simulink model "SP_nonlinear_LQR"  (R2016b)
settings: Solver=ode4  StartTime=0.0  StopTime=100  FixedStep=0.001  RelTol=1e-3
values from neighbouring files (symbols this model uses):
  K = lqr(P_sp,Q,R)    [SP_LQG_controller_design.m]
  Ke_sp = K_bar(:,1)    [SP_LQG_controller_design.m]    (also in controller_parameter.mat = -14.1421356237)
  Kx_sp = K_bar(:,2:end)    [SP_LQG_controller_design.m]    (also in controller_parameter.mat = [-9.4028503548 -29.2130812278])
undefined symbols (not defined in the file or in its folder): An, Aqw, Asp1, Bn, Bqw, Bsp1, Cn, Cqw, Csp1, Kn, lin_sys, Nu, Nu_inv, Nx, Ny, op
libraries: aerolibatmos2 x10, aerolib3dof2 x1, aerolib6dof2 x1, aerolibasang x1
(part 1 of 7)
settings Model: Creator=whn  LastModifiedBy=whn

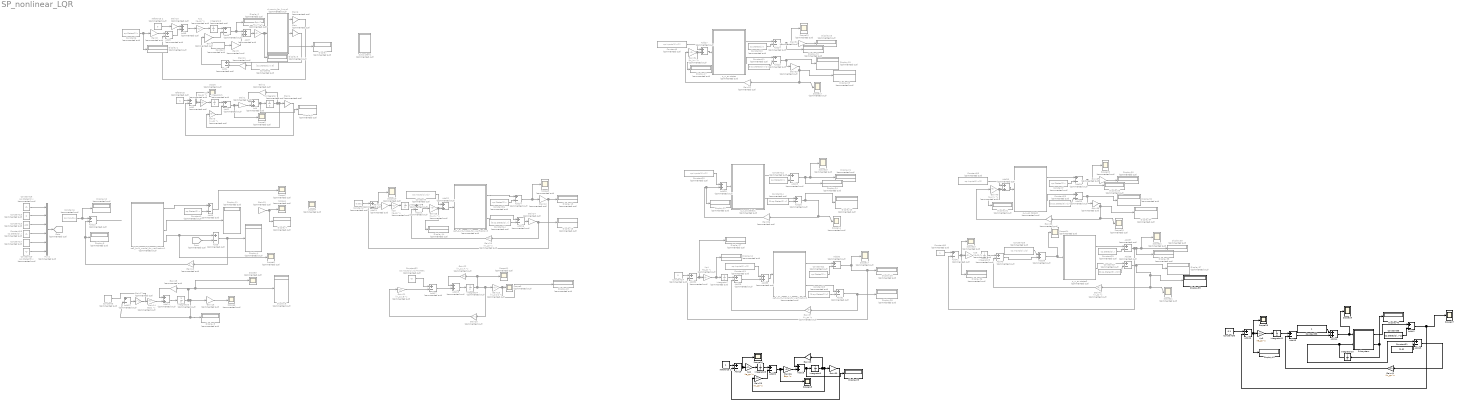
== system SP_nonlinear_LQR ==
  Add{,5,7,11,15,22,27..28,33,36,39} (11 alike) : Sum  Commented=on
  Add{1..4,6,8..10,12..14,16..17,21,23..26,29..32,34..35,37..38,40..41} (28 alike) : Sum  Commented=on  Inputs=+-
  Add18 : Sum
  Add{19..20,42..43,45..46} (6 alike) : Sum  Inputs=+-
  Add44 : Sum
  Constant : Constant  Commented=on  Value=op.Inputs.u(2)
  Constant{1,6..7,10,12,16,18,22,29,34} (10 alike) : Constant  Commented=on  Value=op.States(2).x
  Constant11 : Constant  Commented=on  Value=[0;op.States(3).x(2)]
  Constant13 : Constant  Commented=on  Value=400
  Constant14 : Constant  Commented=on  Value=[0;op.States(2).x]
  Constant15 : Constant  Commented=on  Value=0
  Constant17 : Constant  Commented=on  Value=10000
  Constant19 : Constant  Commented=on  Value=op.States(5).x
  Constant2 : Constant  Commented=on  Value=[op.States(2).x;0]
  Constant{3,9,20..21,26,28} (6 alike) : Constant  Commented=on  Value=op.Inputs(1).u(2)
  Constant23 : Constant  Commented=on  Value=[0;op.States(2).x]
  Constant24 : Constant  Commented=on  Value=0
  Constant25 : Constant  Commented=on  Value=[0;op.States(3).x(2)]
  Constant27 : Constant  Commented=on  Value=[0;op.States(3).x(2)]
  Constant30 : Constant  Commented=on
  Constant31 : Constant  Value=[1;0]  VectorParams1D=off
  Constant32 : Constant  Commented=on  Value=op.Inputs(1).u(2)*0.0001
  Constant33 : Constant
  Constant35 : Constant  Value=op.States(2).x*10
  Constant36 : Constant  Value=0.1
  Constant4 : Constant  Commented=on  Value=op.Inputs.u
  Constant44 : Constant  Commented=on  Value=[0;op.States(2).x]
  Constant5 : Constant  Commented=on  Value=[0 0.001]
  Constant8 : Constant  Commented=on  Value=0.001
  Display{,1..28,30..38} (38 alike) : Display  Commented=on
  Display{29,39..41} (4 alike) : Display
  From : From  Commented=on  GotoTag=states0
  Gain{,11,13,24,33,39} (6 alike) : Gain  Commented=on  Gain=Nx  Multiplication=Matrix(K*u)
  Gain1 : Gain  Commented=on  Gain=Bn  Multiplication=Matrix(K*u)
  Gain{6,8,10,12,27,31,35} (7 alike) : Gain  Commented=on  Gain=Ny  Multiplication=Matrix(K*u)
  Gain14 : Gain  Commented=on  Gain=Bsp1  Multiplication=Matrix(K*u)
  Gain15 : Gain  Commented=on  Gain=Asp1  Multiplication=Matrix(K*u)
  Gain16 : Gain  Commented=on  Gain=Csp1  Multiplication=Matrix(K*u)
  Gain17 : Gain  Commented=on  Gain=K  Multiplication=Matrix(K*u)
  Gain18 : Gain  Commented=on  Gain=K  Multiplication=Matrix(K*u)
  Gain{3,5,19,37,42} (5 alike) : Gain  Commented=on  Gain=Kx_sp  Multiplication=Matrix(K*u)
  Gain2 : Gain  Commented=on  Gain=An  Multiplication=Matrix(K*u)
  Gain20 : Gain  Commented=on  Gain=K  Multiplication=Matrix(K*u)
  Gain21 : Gain  Commented=on  Gain=lin_sys.B  Multiplication=Matrix(K*u)
  Gain22 : Gain  Commented=on  Gain=lin_sys.A  Multiplication=Matrix(K*u)
  Gain23 : Gain  Commented=on  Gain=lin_sys.C  Multiplication=Matrix(K*u)
  Gain{7,25,34,40} (4 alike) : Gain  Commented=on  Gain=Nu_inv  Multiplication=Matrix(K*u)
  Gain26 : Gain  Gain=Bqw  Multiplication=Matrix(K*u)
  Gain28 : Gain  Gain=Aqw  Multiplication=Matrix(K*u)
  Gain29 : Gain  Gain=Kx_sp  Multiplication=Matrix(K*u)
  Gain30 : Gain  Gain=Cqw  Multiplication=Matrix(K*u)
  Gain32 : Gain  Commented=on  Gain=-Kn  Multiplication=Matrix(K*u)
  Gain36 : Gain  Commented=on  Gain=-K  Multiplication=Matrix(K*u)
  Gain38 : Gain  Commented=on  Gain=-Kn  Multiplication=Matrix(K*u)
  Gain4 : Gain  Commented=on  Gain=Cn  Multiplication=Matrix(K*u)
  Gain41 : Gain  Gain=Kx_sp  Multiplication=Matrix(K*u)
  Gain9 : Gain  Commented=on  Gain=Nu  Multiplication=Matrix(K*u)
  Goto : Goto  Commented=on  GotoTag=states0
  Integrator{,1..4,6..7,9} (8 alike) : Integrator  Commented=on
  Integrator10 : Integrator  InitialCondition=[1;0]
  Integrator11 : Integrator
  Integrator5 : Integrator
  Integrator8 : Integrator
  Kp{,1,3..4,6} (5 alike) : Gain  Commented=on  Gain=Ke_sp  Multiplication=Matrix(K*u)
  Kp2 : Gain  Gain=Ke_sp  Multiplication=Matrix(K*u)
  Kp5 : Gain  Gain=Ke_sp  Multiplication=Matrix(K*u)
  Mux2 : Mux  Commented=on  Inputs=6
  Scope{,1..15,17,19..24} (23 alike) : Scope  Commented=on
  Scope{16,18,27..29} (5 alike) : Scope
  Subsystem : Subsystem
  Subsystem1 : Subsystem  Commented=on
  dynamic_for_linsys1 : Subsystem  Commented=on
  q_w_as states : Subsystem  Commented=on
  q_w_as states1 : Subsystem  Commented=on
  q_w_as states2 : Subsystem  Commented=on
  q_w_as states3 : Subsystem  Commented=on
  "reference " : Constant  Commented=on
  reference 1 : Constant
  reference 2 : Constant  Commented=on  Value=0
  sefl_built_model_for_verification1 : Subsystem  Commented=on
  sefl_built_model_for_verification2 : Subsystem  Commented=on
  sefl_built_model_for_verification3 : Subsystem  Commented=on
  wires:
  Gain1/1 -> Add/2
  Add/1 -> Display5/1, Integrator/1
  Gain2/1 -> Add/1
  Gain3/1 -> Add2/2
  Integrator/1 -> Gain3/1, Gain4/1, Gain2/1
  Constant/1 -> Gain9/1
  Gain5/1 -> Add6/2
  Add7/1 -> Gain7/1
  Constant2/1 -> Gain11/1
  Add4/1 -> Gain5/1
  Gain4/1 -> Add1/2
  Add1/1 -> Scope/1, Kp/1
  Kp/1 -> Integrator1/1
  "reference "/1 -> Add1/1
  Integrator1/1 -> Add2/1
  Add2/1 -> Scope2/1, Gain1/1
  Kp1/1 -> Integrator2/1
  Integrator2/1 -> Add6/1
  Add6/1 -> Display2/1, Add7/1
  Constant6/1 -> Display1/1, Gain8/1
  Gain6/1 -> Add3/2
  reference 2/1 -> Gain10/1
  Add3/1 -> Add5/2
  Add5/1 -> Kp1/1
  dynamic_for_linsys1/3(states_dot) -> Display/1
  dynamic_for_linsys1/2("states ") -> Gain/1
  Gain/1 -> Add4/1
  dynamic_for_linsys1/1(output_alpha) -> Gain6/1
  Gain7/1 -> Display3/1, dynamic_for_linsys1/1(In1)
  Gain8/1 -> Add3/1
  Gain9/1 -> Add7/2
  Gain10/1 -> Add5/1
  Gain11/1 -> Add4/2
  sefl_built_model_for_verification1/1(Out5) -> Add8/1
  Constant4/1 -> Display10/1, Add13/1
  Constant1/1 -> Add8/2
  Add8/1 -> Scope7/1
  Add9/1 -> Gain18/1, Display4/1
  sefl_built_model_for_verification1/4(states) -> Add9/1, Scope8/1
  Gain13/1 -> Scope1/1, Display7/1
  Gain14/1 -> Add11/2
  Add11/1 -> Integrator3/1
  Gain15/1 -> Add11/1
  Integrator3/1 -> Display8/1, Add12/2, Gain16/1, Scope3/1, Display6/1, Gain15/1
  Gain18/1 -> Add13/2, Display9/1
  Add12/1 -> Gain17/1
  Constant5/1 -> Gain14/1
  Gain17/1 -> ?
  Gain16/1 -> Scope6/1
  Constant13/1 -> Mux2/3
  Constant16/1 -> Mux2/1
  Constant15/1 -> Mux2/2
  Constant18/1 -> Mux2/4
  Constant17/1 -> Mux2/5
  Constant19/1 -> Mux2/6
  Mux2/1 -> Goto/1
  From/1 -> Add9/2
  Add13/1 -> ?
  sefl_built_model_for_verification1/3(states_dot) -> Display11/1
  Add15/1 -> Integrator4/1
  Gain22/1 -> Add15/1
  Integrator4/1 -> Gain20/1, Gain23/1, Scope11/1, Gain22/1
  Constant32/1 -> Add17/1
  Constant3/1 -> Add22/1
  sefl_built_model_for_verification3/1(alpha_for_tracking) -> Add14/1
  Constant34/1 -> Add14/2
  Add14/1 -> Scope5/1, Gain12/1
  Gain23/1 -> Display18/1, Scope9/1
  sefl_built_model_for_verification3/2(states_q_w) -> Add16/1
  Constant44/1 -> Add16/2
  Gain24/1 -> Gain19/1, Display15/1
  Gain19/1 -> Add10/2
  Gain20/1 -> Gain21/1
  Gain21/1 -> Add17/2
  Add17/1 -> Add15/2
  Add16/1 -> Gain24/1
  Gain25/1 -> Display14/1, Add22/2
  Integrator6/1 -> Add10/1
  Kp3/1 -> Integrator6/1
  Add21/1 -> Scope10/1, Gain27/1
  Gain27/1 -> Kp3/1
  Gain12/1 -> Display13/1, Add21/2  "tracking design for normalized system"
  Constant8/1 -> Add21/1
  Add10/1 -> Gain25/1
  Add22/1 -> sefl_built_model_for_verification3/1(In1)
  Constant9/1 -> Add27/1
  q_w_as states/1(alpha_for_tracking) -> Add24/1
  Constant10/1 -> Add24/2
  Add24/1 -> Display20/1, Scope13/1, Gain31/1
  q_w_as states/2(states_q_w) -> Add25/1
  Constant11/1 -> Add25/2
  Gain33/1 -> Display25/1, Scope12/1, Gain32/1  "normalized system for lqr verification"
  Gain32/1 -> Gain34/1
  Add25/1 -> Gain33/1, Display19/1
  Gain34/1 -> Display17/1, Add27/2
  Gain31/1 -> Display16/1
  Add27/1 -> q_w_as states/1(In1)
  Constant20/1 -> Add28/1
  q_w_as states1/1(alpha_for_tracking) -> Add23/1
  Constant12/1 -> Add23/2
  q_w_as states1/2(states_q_alpha) -> Add26/1
  Constant14/1 -> Add26/2
  Add26/1 -> Scope14/1, Gain36/1, Display23/1  "non_normalized system for lqr verification"
  Gain36/1 -> Add28/2, Display22/1
  Add23/1 -> Display24/1, Display21/1, Scope15/1
  Add28/1 -> q_w_as states1/1(In1)
  Constant21/1 -> Add33/1
  sefl_built_model_for_verification2/1(alpha_for_tracking) -> Add30/1
  Constant22/1 -> Add30/2
  sefl_built_model_for_verification2/2(states_q_alpha) -> Add31/1
  Constant23/1 -> Add31/2
  Add31/1 -> Gain37/1, Display28/1
  Gain37/1 -> Add29/2
  Add29/1 -> Add33/2
  Integrator7/1 -> Add29/1
  Kp4/1 -> Display12/1, Integrator7/1
  Add32/1 -> Display27/1, Kp4/1
  Add30/1 -> Display26/1, Add32/2, Scope17/1  "non-normalized system for tracking"
  Constant24/1 -> Add32/1
  Add33/1 -> sefl_built_model_for_verification2/1(In1)
  Gain26/1 -> Add18/2
  Add18/1 -> Integrator5/1, Display29/1
  Gain28/1 -> Add18/1
  Gain29/1 -> Add20/2
  Integrator5/1 -> Gain28/1, Gain30/1, Gain29/1
  Gain30/1 -> Add19/2
  Add19/1 -> Kp2/1, Scope16/1
  Kp2/1 -> Integrator8/1
  reference 1/1 -> Add19/1
  Integrator8/1 -> Add20/1
  Add20/1 -> Gain26/1, Scope18/1
  Constant26/1 -> Add36/1
  q_w_as states2/1(alpha_for_tracking) -> Add34/1
  Constant7/1 -> Add34/2
  Add34/1 -> Display33/1, Scope20/1, Gain35/1
  q_w_as states2/2(states_q_w) -> Add35/1
  Constant25/1 -> Add35/2
  Gain39/1 -> Display34/1, Scope19/1, Gain38/1  "normalized system for lqr verification_q_w"
  Gain38/1 -> Gain40/1
  Add35/1 -> Gain39/1, Display32/1
  Gain40/1 -> Display31/1, Add36/2
  Gain35/1 -> Display30/1
  Add36/1 -> q_w_as states2/1(In1)
  Constant28/1 -> Add39/1
  q_w_as states3/1(alpha_for_tracking) -> Add37/1
  Constant29/1 -> Add37/2
  q_w_as states3/2(states_q_w) -> Add38/1
  Constant27/1 -> Add38/2
  Add38/1 -> Display39/1, Scope21/1, Gain42/1, Display37/1  "non_normalized system for lqr verification_q_W"
  Add39/1 -> q_w_as states3/1(In1), Scope24/1
  Gain42/1 -> Add40/2
  Add40/1 -> Add39/2
  Integrator9/1 -> Add40/1
  Kp6/1 -> Integrator9/1
  Add41/1 -> Display36/1, Scope23/1, Kp6/1
  Add37/1 -> Display38/1, Display35/1, Scope22/1, Add41/2  "non-normalized system for tracking"
  Constant30/1 -> Add41/1
  Subsystem/2(Xdotbar) -> Integrator10/1, Display40/1
  Integrator10/1 -> Subsystem/2(Xbar), Add43/1
  Constant33/1 -> Add44/1
  Subsystem/1(Ybar) -> Add42/1
  Constant35/1 -> Add42/2
  Constant31/1 -> Add43/2
  Add43/1 -> Gain41/1
  Add44/1 -> Scope29/1, Subsystem/1(Ubar)
  Gain41/1 -> Add45/2
  Add45/1 -> Add44/2
  Integrator11/1 -> Add45/1
  Kp5/1 -> Integrator11/1
  Add46/1 -> Display41/1, Scope28/1, Kp5/1
  Add42/1 -> Scope27/1, Add46/2  "non-normalized system for tracking"
  Constant36/1 -> Add46/1

== system SP_nonlinear_LQR/Subsystem ==
  Ubar : Inport
  Xbar : Inport  Port=2
  Constant2 : Constant  Value=10
  Constant24 : Constant
  Constant25 : Constant  Value=op.States(3).x(2)
  Constant29 : Constant  Value=op.Inputs(1).u(2)
  Demux3 : Demux  Outputs=2
  Mux3 : Mux  Inputs=2
  Product : Product  Inputs=*/
  Product1 : Product
  Product2 : Product
  Product3 : Product
  sefl_built_model : Subsystem
  Ybar : Outport
  Xdotbar : Outport  Port=2
  wires:
  Mux3/1 -> Product/2, Product3/1
  Xbar/1 -> Product3/2
  sefl_built_model/1(alpha_for_tracking) -> Product1/1
  Product1/1 -> Ybar/1
  Product3/1 -> Demux3/1
  sefl_built_model/2(states_dot) -> Product/1
  Constant29/1 -> Product2/1
  Constant2/1 -> Product1/2
  Product2/1 -> sefl_built_model/1(In1)
  Product/1 -> Xdotbar/1
  Demux3/1 -> sefl_built_model/2(w)
  Constant25/1 -> Mux3/1
  Constant24/1 -> Mux3/2
  Demux3/2 -> sefl_built_model/3(q)
  Ubar/1 -> Product2/2

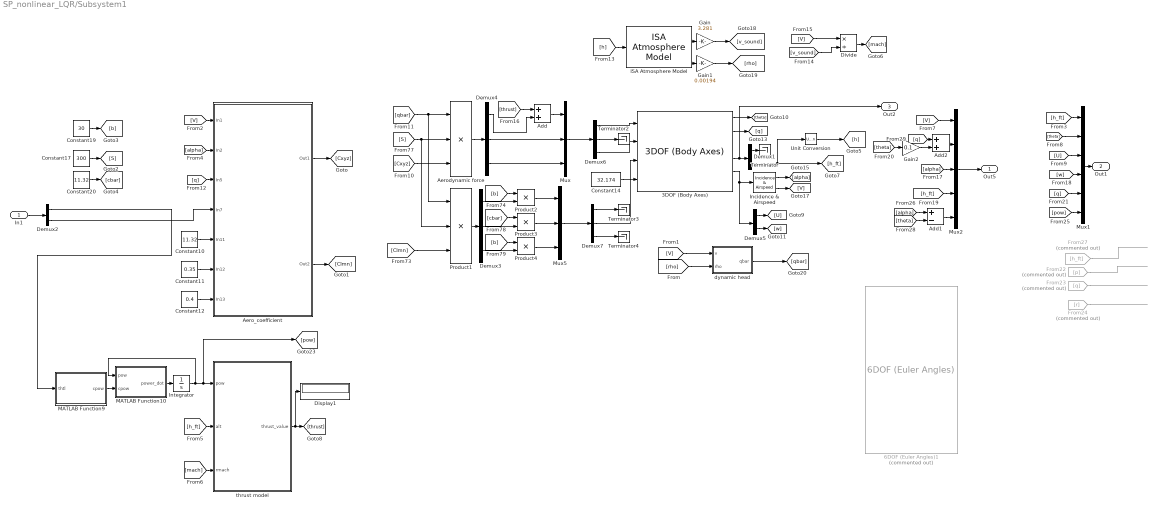
== system SP_nonlinear_LQR/Subsystem1 ==
  In1 : Inport
  3DOF (Body Axes) : aerolib3dof2/3DOF (Body Axes)  units=English (Velocity in ft/s)  mtype=Fixed  v_ini=400  theta_ini=op.States(2).x  alpha_ini=op.States(2).x  q_ini=0  pos_ini=[0 10000]  mass=1/1.57e-3  mass_e=0.5  mass_f=3.0  Iyy=55814  Iyy_e=0.5  Iyy_f=3.0  g_in=External  g=9.81  vre_flag=on
  6DOF (Euler Angles)1 : aerolib6dof2/6DOF (Euler Angles)  Commented=on  units=English (Velocity in ft/s)  mtype=Fixed  rep=Euler Angles  xme_0=[0 0 10000]  Vm_0=[294.1676 0.0066 58.8681]  eul_0=[0 0.1975 0]  pm_0=[0 0 0]  mass_0=1/1.57e-3  mass_e=0.5  mass_f=2.0  inertia=[9496 0 -982;0 55814 0;0 0 63100]  inertia_e=eye(3)  inertia_f=2*eye(3)  k_quat=1.0  vre_flag=on
  Add : Sum
  Add1 : Sum  Inputs=+-
  Add2 : Sum
  Aero_coefficient : Subsystem
      mask Display:
      | port_label('input', 1, 'vt')
      | port_label('input', 2, 'alpha')
      | 
      | port_label('input', 3, 'q')
      | 
      | port_label('input', 4, 'el')
      | 
      | 
      | 
      | port_label('input', 5, 'cbar')
      | port_label('input', 6, 'xcgr')
      | port_label('input', 7, 'xcg')
      | port_label('output', 1, 'Cxz')
      | port_label('output', 2, 'Cm')
  "Aerodynamic force " : Product  Inputs=3
  Constant10 : Constant  Value=11.32
  Constant11 : Constant  Value=0.35
  Constant12 : Constant  Value=0.4
  Constant14 : Constant  Value=32.174
  Constant17 : Constant  Value=300
  Constant19 : Constant  Value=30
  Constant20 : Constant  Value=11.32
  Demux1 : Demux  Outputs=2
  Demux2 : Demux  Outputs=2
  Demux{3..4,6..7} (4 alike) : Demux  Outputs=3
  Demux5 : Demux  Outputs=2
  Display1 : Display
  Divide : Product  Inputs=*/
  From22 : From  Commented=on  GotoTag=p
  From23 : From  Commented=on  GotoTag=q
  From24 : From  Commented=on  GotoTag=r
  From27 : From  Commented=on  GotoTag=h_ft
  Gain : Gain  Gain=3.281
  Gain1 : Gain  Gain=0.00194
  Gain2 : Gain  Gain=0.1
  ISA Atmosphere Model : aerolibatmos2/ISA Atmosphere Model  custom=off  g=9.80665  gamma=1.4  R=287.0531  L=0.0065  h_trop=11000  h_strat=20000  rho0=1.225  P0=101325  T0=288.15  h0=0
  Incidence & Airspeed : aerolibasang/Incidence  & Airspeed
  Integrator : Integrator  InitialCondition=op.states(5).x
  MATLAB Function10 : MATLAB Function  TreatAsAtomicUnit=on
  MATLAB Function9 : MATLAB Function  TreatAsAtomicUnit=on
  Mux : Mux  Inputs=3
  Mux1 : Mux  Inputs=6
  Mux2 : Mux  Inputs=5
  Mux5 : Mux  Inputs=3
  Product1 : Product  Inputs=3
  Product2 : Product
  Product3 : Product
  Product4 : Product
  Terminator{,2..4} (4 alike) : Terminator
  Unit Conversion : UnitConversion
  dynamic head : MATLAB Function  TreatAsAtomicUnit=on
  thrust model : MATLAB Function  TreatAsAtomicUnit=on
  Out5 : Outport
  Out1 : Outport  Port=2
  Out2 : Outport  Port=3
  wires:
  Add2/1 -> Mux2/2
  Gain2/1 -> Add2/2
  [q] -> Add2/1
  [theta] -> Add1/2
  [alpha] -> Add1/1
  Add1/1 -> Mux2/5
  3DOF (Body Axes)/5 -> Demux5/1, Incidence & Airspeed/1
  Mux2/1 -> Out5/1
  Incidence & Airspeed/2 -> [V]
  3DOF (Body Axes)/4 -> Demux1/1, Out2/1
  ISA Atmosphere Model/4 -> Gain1/1
  ISA Atmosphere Model/2 -> Gain/1
  [qbar] -> Product1/1, "Aerodynamic force "/1
  In1/1 -> Demux2/1
  Product4/1 -> Mux5/3
  Constant10/1 -> Aero_coefficient/5(In11)
  Constant11/1 -> Aero_coefficient/6(In12)
  Mux5/1 -> Demux7/1
  Constant17/1 -> [S]
  [q] -> Aero_coefficient/3(In5)
  Gain1/1 -> [rho]
  Product3/1 -> Mux5/2
  Product2/1 -> Mux5/1
  [V] -> Divide/1
  [V] -> dynamic head/1(v)
  Aero_coefficient/1(Out1) -> [Cxyz]
  [rho] -> dynamic head/2(rho)
  Aero_coefficient/2(Out2) -> [Clmn]
  Constant20/1 -> [cbar]
  Constant19/1 -> [b]
  Demux1/2 -> [h_ft], Unit Conversion/1
  [h] -> ISA Atmosphere Model/1
  Demux4/3 -> Mux/3
  Gain/1 -> [v_sound]
  Divide/1 -> [mach]
  Add/1 -> Mux/1
  Demux4/2 -> Mux/2
  [v_sound] -> Divide/2
  Demux4/1 -> Add/2
  Mux/1 -> Demux6/1
  Constant12/1 -> Aero_coefficient/7(In13)
  [alpha] -> Aero_coefficient/2(In2)
  Unit Conversion/1 -> [h]
  dynamic head/1(qbar) -> [qbar]
  thrust model/1(thrust_value) -> Display1/1, [thrust]
  Incidence & Airspeed/1 -> [alpha]
  [h_ft] -> thrust model/2(alt)
  Demux2/2 -> Aero_coefficient/4(In7)
  Demux2/1 -> MATLAB Function9/1(thtl)
  Integrator/1 -> MATLAB Function10/1(pow), [pow], thrust model/1(pow)
  [mach] -> thrust model/3(rmach)
  [alpha] -> Mux2/3
  MATLAB Function10/1(power_dot) -> Integrator/1
  [V] -> Aero_coefficient/1(In1)
  MATLAB Function9/1(cpow) -> MATLAB Function10/2(cpow)
  [thrust] -> Add/1
  Demux3/3 -> Product4/2
  [b] -> Product4/1
  "Aerodynamic force "/1 -> Demux4/1
  [Cxyz] -> "Aerodynamic force "/3
  [S] -> "Aerodynamic force "/2, Product1/2
  [Clmn] -> Product1/3
  [b] -> Product2/1
  Product1/1 -> Demux3/1
  Demux3/1 -> Product2/2
  Demux3/2 -> Product3/2
  [cbar] -> Product3/1
  [theta] -> Gain2/1
  [V] -> Mux2/1
  From27/1 -> ?
  From22/1 -> ?
  From23/1 -> ?
  From24/1 -> ?
  [h_ft] -> Mux2/4
  Demux6/1 -> 3DOF (Body Axes)/1
  Demux6/3 -> 3DOF (Body Axes)/2
  Demux6/2 -> Terminator2/1
  Demux7/2 -> 3DOF (Body Axes)/3
  Demux7/1 -> Terminator3/1
  Demux7/3 -> Terminator4/1
  Demux1/1 -> Terminator/1
  3DOF (Body Axes)/1 -> [theta]
  3DOF (Body Axes)/2 -> [q]
  Constant14/1 -> 3DOF (Body Axes)/4
  [h_ft] -> Mux1/1
  [theta] -> Mux1/2
  Demux5/2 -> [w]
  Demux5/1 -> [U]
  [U] -> Mux1/3
  [w] -> Mux1/4
  [q] -> Mux1/5
  [pow] -> Mux1/6
  Mux1/1 -> Out1/1

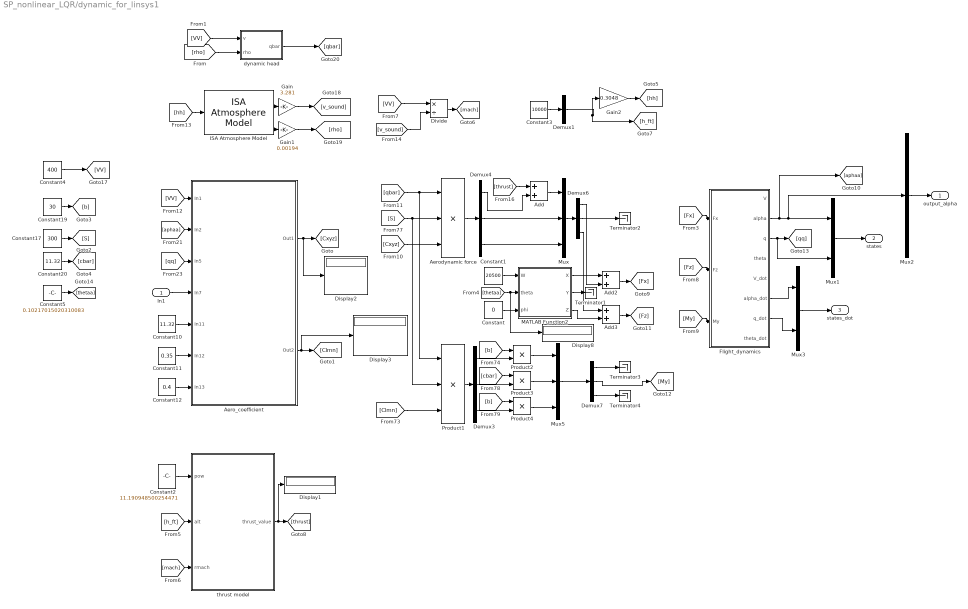
== system SP_nonlinear_LQR/dynamic_for_linsys1 ==
  In1 : Inport
  Add : Sum
  Add2 : Sum
  Add3 : Sum
  Aero_coefficient : Subsystem
      mask Display:
      | port_label('input', 1, 'vt')
      | port_label('input', 2, 'alpha')
      | 
      | port_label('input', 3, 'q')
      | 
      | port_label('input', 4, 'el')
      | 
      | 
      | 
      | port_label('input', 5, 'cbar')
      | port_label('input', 6, 'xcgr')
      | port_label('input', 7, 'xcg')
      | port_label('output', 1, 'Cxz')
      | port_label('output', 2, 'Cm')
  "Aerodynamic force " : Product  Inputs=3
  Constant : Constant  Value=0
  Constant1 : Constant  Value=20500
  Constant10 : Constant  Value=11.32
  Constant11 : Constant  Value=0.35
  Constant12 : Constant  Value=0.4
  Constant17 : Constant  Value=300
  Constant19 : Constant  Value=30
  Constant2 : Constant  Value=11.190948500254471
  Constant20 : Constant  Value=11.32
  Constant3 : Constant  Value=10000
  Constant4 : Constant  Value=400
  Constant5 : Constant  Value=0.10217015020310083
  Demux1 : Demux  Outputs=1
  Demux{3..4,6..7} (4 alike) : Demux  Outputs=3
  Display{1..3,8} (4 alike) : Display
  Divide : Product  Inputs=*/
  Flight_dynamics : Subsystem
  Gain : Gain  Gain=3.281
  Gain1 : Gain  Gain=0.00194
  Gain2 : Gain  Gain=0.3048
  ISA Atmosphere Model : aerolibatmos2/ISA Atmosphere Model  custom=off  g=9.80665  gamma=1.4  R=287.0531  L=0.0065  h_trop=11000  h_strat=20000  rho0=1.225  P0=101325  T0=288.15  h0=0
  MATLAB Function2 : MATLAB Function  TreatAsAtomicUnit=on
  Mux : Mux  Inputs=3
  Mux1 : Mux  Inputs=2
  Mux2 : Mux  Inputs=1
  Mux3 : Mux  Inputs=2
  Mux5 : Mux  Inputs=3
  Product1 : Product  Inputs=3
  Product2 : Product
  Product3 : Product
  Product4 : Product
  Terminator{1..4} (4 alike) : Terminator
  dynamic head : MATLAB Function  TreatAsAtomicUnit=on
  thrust model : MATLAB Function  TreatAsAtomicUnit=on
  output_alpha : Outport
  "states " : Outport  Port=2
  states_dot : Outport  Port=3
  wires:
  [qq] -> Aero_coefficient/3(In5)
  [aphaa] -> Aero_coefficient/2(In2)
  [VV] -> Aero_coefficient/1(In1)
  Constant5/1 -> [thetaa]
  Flight_dynamics/3(q) -> Mux1/2, [qq]
  Flight_dynamics/2(alpha) -> [aphaa], Mux1/1, Mux2/1
  ISA Atmosphere Model/4 -> Gain1/1
  ISA Atmosphere Model/2 -> Gain/1
  [qbar] -> Product1/1, "Aerodynamic force "/1
  In1/1 -> Aero_coefficient/4(In7)
  Product4/1 -> Mux5/3
  Constant10/1 -> Aero_coefficient/5(In11)
  Constant11/1 -> Aero_coefficient/6(In12)
  Mux5/1 -> Demux7/1
  Constant17/1 -> [S]
  Gain1/1 -> [rho]
  Product3/1 -> Mux5/2
  Product2/1 -> Mux5/1
  [VV] -> Divide/1
  [VV] -> dynamic head/1(v)
  Aero_coefficient/1(Out1) -> Display2/1, [Cxyz]
  [rho] -> dynamic head/2(rho)
  Aero_coefficient/2(Out2) -> Display3/1, [Clmn]
  Constant20/1 -> [cbar]
  Constant19/1 -> [b]
  Demux1/1 -> [h_ft], Gain2/1
  [hh] -> ISA Atmosphere Model/1
  Demux4/3 -> Mux/3
  Gain/1 -> [v_sound]
  Divide/1 -> [mach]
  Add/1 -> Mux/1
  Demux4/2 -> Mux/2
  [v_sound] -> Divide/2
  Demux4/1 -> Add/2
  Mux/1 -> Demux6/1
  Constant12/1 -> Aero_coefficient/7(In13)
  Gain2/1 -> [hh]
  dynamic head/1(qbar) -> [qbar]
  thrust model/1(thrust_value) -> Display1/1, [thrust]
  [h_ft] -> thrust model/2(alt)
  [mach] -> thrust model/3(rmach)
  Constant4/1 -> [VV]
  [thrust] -> Add/1
  Demux3/3 -> Product4/2
  [b] -> Product4/1
  "Aerodynamic force "/1 -> Demux4/1
  [Cxyz] -> "Aerodynamic force "/3
  [S] -> "Aerodynamic force "/2, Product1/2
  [Clmn] -> Product1/3
  [b] -> Product2/1
  Product1/1 -> Demux3/1
  Demux3/1 -> Product2/2
  Demux3/2 -> Product3/2
  [cbar] -> Product3/1
  Demux6/3 -> Add3/1
  Demux6/2 -> Terminator2/1
  Demux7/1 -> Terminator3/1
  Demux7/3 -> Terminator4/1
  Mux2/1 -> output_alpha/1
  Constant1/1 -> MATLAB Function2/1(W)
  [thetaa] -> Display8/1, MATLAB Function2/2(theta)
  Constant/1 -> MATLAB Function2/3(phi)
  MATLAB Function2/1(X) -> Add2/1
  Demux6/1 -> Add2/2
  MATLAB Function2/3(Z) -> Add3/2
  MATLAB Function2/2(Y) -> Terminator1/1
  Add2/1 -> [Fx]
  Add3/1 -> [Fz]
  Demux7/2 -> [My]
  [Fx] -> Flight_dynamics/1(Fx)
  [Fz] -> Flight_dynamics/2(Fz)
  [My] -> Flight_dynamics/3(My)
  Mux1/1 -> "states "/1
  Flight_dynamics/6(alpha_dot) -> Mux3/1
  Flight_dynamics/7(q_dot) -> Mux3/2
  Mux3/1 -> states_dot/1
  Constant2/1 -> thrust model/1(pow)
  Constant3/1 -> Demux1/1

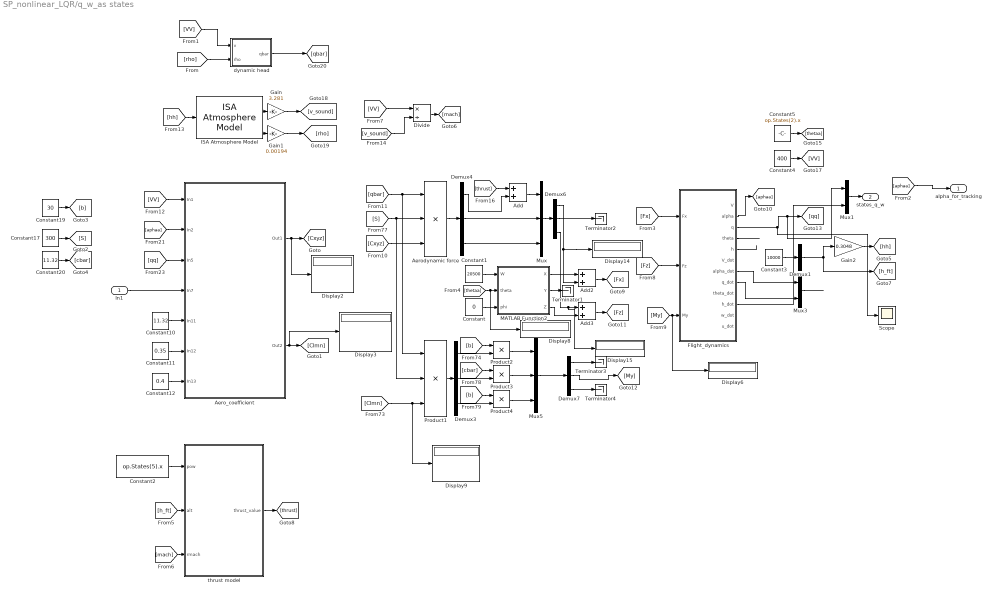
== system SP_nonlinear_LQR/q_w_as states ==
  In1 : Inport
  Add : Sum
  Add2 : Sum
  Add3 : Sum
  Aero_coefficient : Subsystem
      mask Display:
      | port_label('input', 1, 'vt')
      | port_label('input', 2, 'alpha')
      | 
      | port_label('input', 3, 'q')
      | 
      | port_label('input', 4, 'el')
      | 
      | 
      | 
      | port_label('input', 5, 'cbar')
      | port_label('input', 6, 'xcgr')
      | port_label('input', 7, 'xcg')
      | port_label('output', 1, 'Cxz')
      | port_label('output', 2, 'Cm')
  "Aerodynamic force " : Product  Inputs=3
  Constant : Constant  Value=0
  Constant1 : Constant  Value=20500
  Constant10 : Constant  Value=11.32
  Constant11 : Constant  Value=0.35
  Constant12 : Constant  Value=0.4
  Constant17 : Constant  Value=300
  Constant19 : Constant  Value=30
  Constant2 : Constant  Value=op.States(5).x
  Constant20 : Constant  Value=11.32
  Constant3 : Constant  Value=10000
  Constant4 : Constant  Value=400
  Constant5 : Constant  Value=op.States(2).x
  Demux1 : Demux  Outputs=1
  Demux{3..4,6..7} (4 alike) : Demux  Outputs=3
  Display{2..3,6,8..9,14..15} (7 alike) : Display
  Divide : Product  Inputs=*/
  Flight_dynamics : Subsystem
  Gain : Gain  Gain=3.281
  Gain1 : Gain  Gain=0.00194
  Gain2 : Gain  Gain=0.3048
  ISA Atmosphere Model : aerolibatmos2/ISA Atmosphere Model  custom=off  g=9.80665  gamma=1.4  R=287.0531  L=0.0065  h_trop=11000  h_strat=20000  rho0=1.225  P0=101325  T0=288.15  h0=0
  MATLAB Function2 : MATLAB Function  TreatAsAtomicUnit=on
  Mux : Mux  Inputs=3
  Mux1 : Mux  Inputs=2
  Mux3 : Mux  Inputs=2
  Mux5 : Mux  Inputs=3
  Product1 : Product  Inputs=3
  Product2 : Product
  Product3 : Product
  Product4 : Product
  Scope : Scope
  Terminator{1..4} (4 alike) : Terminator
  dynamic head : MATLAB Function  TreatAsAtomicUnit=on
  thrust model : MATLAB Function  TreatAsAtomicUnit=on
  alpha_for_tracking : Outport
  states_q_w : Outport  Port=2
  wires:
  [aphaa] -> alpha_for_tracking/1
  Constant5/1 -> [thetaa]
  Constant4/1 -> [VV]
  Constant3/1 -> Demux1/1
  Constant2/1 -> thrust model/1(pow)
  Flight_dynamics/8(q_dot) -> Mux3/2
  Flight_dynamics/7(alpha_dot) -> Mux3/1
  [qq] -> Aero_coefficient/3(In5)
  [aphaa] -> Aero_coefficient/2(In2)
  [VV] -> Aero_coefficient/1(In1)
  Flight_dynamics/5(h) -> ?
  ISA Atmosphere Model/4 -> Gain1/1
  ISA Atmosphere Model/2 -> Gain/1
  [qbar] -> Product1/1, "Aerodynamic force "/1
  In1/1 -> Aero_coefficient/4(In7)
  Product4/1 -> Mux5/3
  Constant10/1 -> Aero_coefficient/5(In11)
  Constant11/1 -> Aero_coefficient/6(In12)
  Mux5/1 -> Demux7/1
  Constant17/1 -> [S]
  Gain1/1 -> [rho]
  Product3/1 -> Mux5/2
  Product2/1 -> Mux5/1
  [VV] -> Divide/1
  [VV] -> dynamic head/1(v)
  Aero_coefficient/1(Out1) -> Display2/1, [Cxyz]
  [rho] -> dynamic head/2(rho)
  Aero_coefficient/2(Out2) -> [Clmn], Display3/1
  Constant20/1 -> [cbar]
  Constant19/1 -> [b]
  Demux1/1 -> Gain2/1, [h_ft]
  [hh] -> ISA Atmosphere Model/1
  Demux4/3 -> Mux/3
  Gain/1 -> [v_sound]
  Divide/1 -> [mach]
  Add/1 -> Mux/1
  Demux4/2 -> Mux/2
  [v_sound] -> Divide/2
  Demux4/1 -> Add/2
  Mux/1 -> Demux6/1
  Constant12/1 -> Aero_coefficient/7(In13)
  Gain2/1 -> [hh]
  dynamic head/1(qbar) -> [qbar]
  thrust model/1(thrust_value) -> [thrust]
  [h_ft] -> thrust model/2(alt)
  [mach] -> thrust model/3(rmach)
  [thrust] -> Add/1
  Demux3/3 -> Product4/2
  [b] -> Product4/1
  "Aerodynamic force "/1 -> Demux4/1
  [Cxyz] -> "Aerodynamic force "/3
  [S] -> "Aerodynamic force "/2, Product1/2
  [Clmn] -> Display9/1, Product1/3
  [b] -> Product2/1
  Product1/1 -> Demux3/1
  Demux3/1 -> Product2/2
  Demux3/2 -> Product3/2
  [cbar] -> Product3/1
  Demux6/3 -> Display15/1, Add3/1
  Demux6/2 -> Terminator2/1
  Demux7/1 -> Terminator3/1
  Demux7/3 -> Terminator4/1
  Constant1/1 -> MATLAB Function2/1(W)
  [thetaa] -> Display8/1, MATLAB Function2/2(theta)
  Constant/1 -> MATLAB Function2/3(phi)
  MATLAB Function2/1(X) -> Add2/1
  Demux6/1 -> Display14/1, Add2/2
  MATLAB Function2/3(Z) -> Add3/2
  MATLAB Function2/2(Y) -> Terminator1/1
  Add2/1 -> [Fx]
  Add3/1 -> [Fz]
  Demux7/2 -> [My]
  [Fx] -> Flight_dynamics/1(Fx)
  [Fz] -> Flight_dynamics/2(Fz)
  [My] -> Flight_dynamics/3(My), Display6/1
  Mux3/1 -> ?
  Flight_dynamics/2(alpha) -> [aphaa]
  Flight_dynamics/3(q) -> Scope/1, Mux1/1, [qq]
  Flight_dynamics/4(theta) -> ?
  Mux1/1 -> states_q_w/1
  Flight_dynamics/10(h_dot) -> Mux1/2

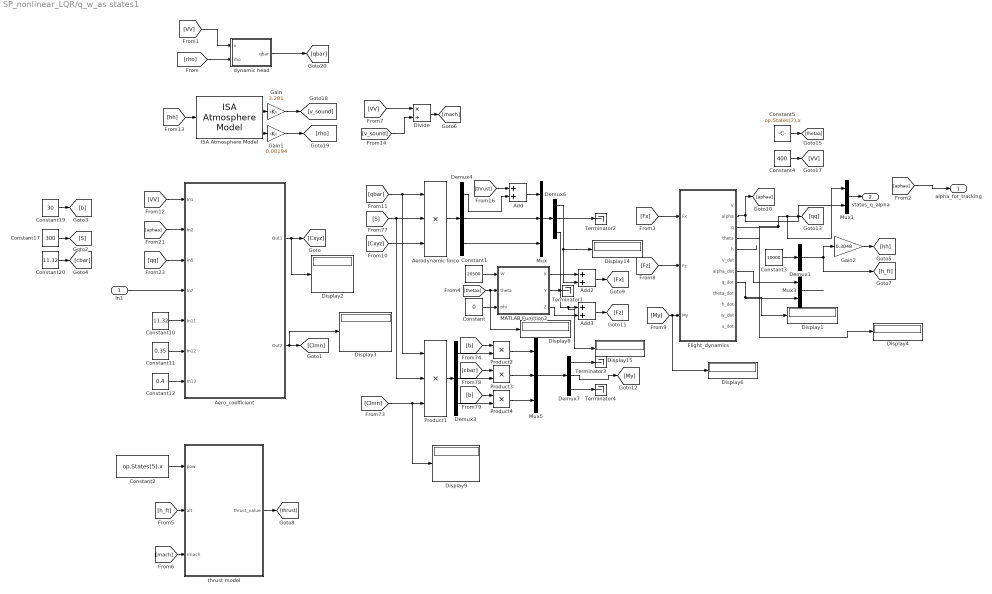
== system SP_nonlinear_LQR/q_w_as states1 ==
  In1 : Inport
  Add : Sum
  Add2 : Sum
  Add3 : Sum
  Aero_coefficient : Subsystem
      mask Display:
      | port_label('input', 1, 'vt')
      | port_label('input', 2, 'alpha')
      | 
      | port_label('input', 3, 'q')
      | 
      | port_label('input', 4, 'el')
      | 
      | 
      | 
      | port_label('input', 5, 'cbar')
      | port_label('input', 6, 'xcgr')
      | port_label('input', 7, 'xcg')
      | port_label('output', 1, 'Cxz')
      | port_label('output', 2, 'Cm')
  "Aerodynamic force " : Product  Inputs=3
  Constant : Constant  Value=0
  Constant1 : Constant  Value=20500
  Constant10 : Constant  Value=11.32
  Constant11 : Constant  Value=0.35
  Constant12 : Constant  Value=0.4
  Constant17 : Constant  Value=300
  Constant19 : Constant  Value=30
  Constant2 : Constant  Value=op.States(5).x
  Constant20 : Constant  Value=11.32
  Constant3 : Constant  Value=10000
  Constant4 : Constant  Value=400
  Constant5 : Constant  Value=op.States(2).x
  Demux1 : Demux  Outputs=1
  Demux{3..4,6..7} (4 alike) : Demux  Outputs=3
  Display{1..4,6,8..9,14..15} (9 alike) : Display
  Divide : Product  Inputs=*/
  Flight_dynamics : Subsystem
  Gain : Gain  Gain=3.281
  Gain1 : Gain  Gain=0.00194
  Gain2 : Gain  Gain=0.3048
  ISA Atmosphere Model : aerolibatmos2/ISA Atmosphere Model  custom=off  g=9.80665  gamma=1.4  R=287.0531  L=0.0065  h_trop=11000  h_strat=20000  rho0=1.225  P0=101325  T0=288.15  h0=0
  MATLAB Function2 : MATLAB Function  TreatAsAtomicUnit=on
  Mux : Mux  Inputs=3
  Mux1 : Mux  Inputs=2
  Mux3 : Mux  Inputs=2
  Mux5 : Mux  Inputs=3
  Product1 : Product  Inputs=3
  Product2 : Product
  Product3 : Product
  Product4 : Product
  Terminator{1..4} (4 alike) : Terminator
  dynamic head : MATLAB Function  TreatAsAtomicUnit=on
  thrust model : MATLAB Function  TreatAsAtomicUnit=on
  alpha_for_tracking : Outport
  states_q_alpha : Outport  Port=2
  wires:
  [aphaa] -> alpha_for_tracking/1
  Constant5/1 -> [thetaa]
  Constant4/1 -> [VV]
  Constant3/1 -> Demux1/1
  Constant2/1 -> thrust model/1(pow)
  Flight_dynamics/8(q_dot) -> Display1/1, Mux3/2
  Flight_dynamics/7(alpha_dot) -> Mux3/1
  [qq] -> Aero_coefficient/3(In5)
  [aphaa] -> Aero_coefficient/2(In2)
  [VV] -> Aero_coefficient/1(In1)
  Flight_dynamics/5(h) -> ?
  ISA Atmosphere Model/4 -> Gain1/1
  ISA Atmosphere Model/2 -> Gain/1
  [qbar] -> Product1/1, "Aerodynamic force "/1
  In1/1 -> Aero_coefficient/4(In7)
  Product4/1 -> Mux5/3
  Constant10/1 -> Aero_coefficient/5(In11)
  Constant11/1 -> Aero_coefficient/6(In12)
  Mux5/1 -> Demux7/1
  Constant17/1 -> [S]
  Gain1/1 -> [rho]
  Product3/1 -> Mux5/2
  Product2/1 -> Mux5/1
  [VV] -> Divide/1
  [VV] -> dynamic head/1(v)
  Aero_coefficient/1(Out1) -> Display2/1, [Cxyz]
  [rho] -> dynamic head/2(rho)
  Aero_coefficient/2(Out2) -> [Clmn], Display3/1
  Constant20/1 -> [cbar]
  Constant19/1 -> [b]
  Demux1/1 -> Gain2/1, [h_ft]
  [hh] -> ISA Atmosphere Model/1
  Demux4/3 -> Mux/3
  Gain/1 -> [v_sound]
  Divide/1 -> [mach]
  Add/1 -> Mux/1
  Demux4/2 -> Mux/2
  [v_sound] -> Divide/2
  Demux4/1 -> Add/2
  Mux/1 -> Demux6/1
  Constant12/1 -> Aero_coefficient/7(In13)
  Gain2/1 -> [hh]
  dynamic head/1(qbar) -> [qbar]
  thrust model/1(thrust_value) -> [thrust]
  [h_ft] -> thrust model/2(alt)
  [mach] -> thrust model/3(rmach)
  [thrust] -> Add/1
  Demux3/3 -> Product4/2
  [b] -> Product4/1
  "Aerodynamic force "/1 -> Demux4/1
  [Cxyz] -> "Aerodynamic force "/3
  [S] -> "Aerodynamic force "/2, Product1/2
  [Clmn] -> Display9/1, Product1/3
  [b] -> Product2/1
  Product1/1 -> Demux3/1
  Demux3/1 -> Product2/2
  Demux3/2 -> Product3/2
  [cbar] -> Product3/1
  Demux6/3 -> Display15/1, Add3/1
  Demux6/2 -> Terminator2/1
  Demux7/1 -> Terminator3/1
  Demux7/3 -> Terminator4/1
  Constant1/1 -> MATLAB Function2/1(W)
  [thetaa] -> Display8/1, MATLAB Function2/2(theta)
  Constant/1 -> MATLAB Function2/3(phi)
  MATLAB Function2/1(X) -> Add2/1
  Demux6/1 -> Display14/1, Add2/2
  MATLAB Function2/3(Z) -> Add3/2
  MATLAB Function2/2(Y) -> Terminator1/1
  Add2/1 -> [Fx]
  Add3/1 -> [Fz]
  Demux7/2 -> [My]
  [Fx] -> Flight_dynamics/1(Fx)
  [Fz] -> Flight_dynamics/2(Fz)
  [My] -> Flight_dynamics/3(My), Display6/1
  Mux3/1 -> ?
  Flight_dynamics/2(alpha) -> Mux1/2, [aphaa]
  Flight_dynamics/3(q) -> Display4/1, Mux1/1, [qq]
  Flight_dynamics/4(theta) -> ?
  Mux1/1 -> states_q_alpha/1

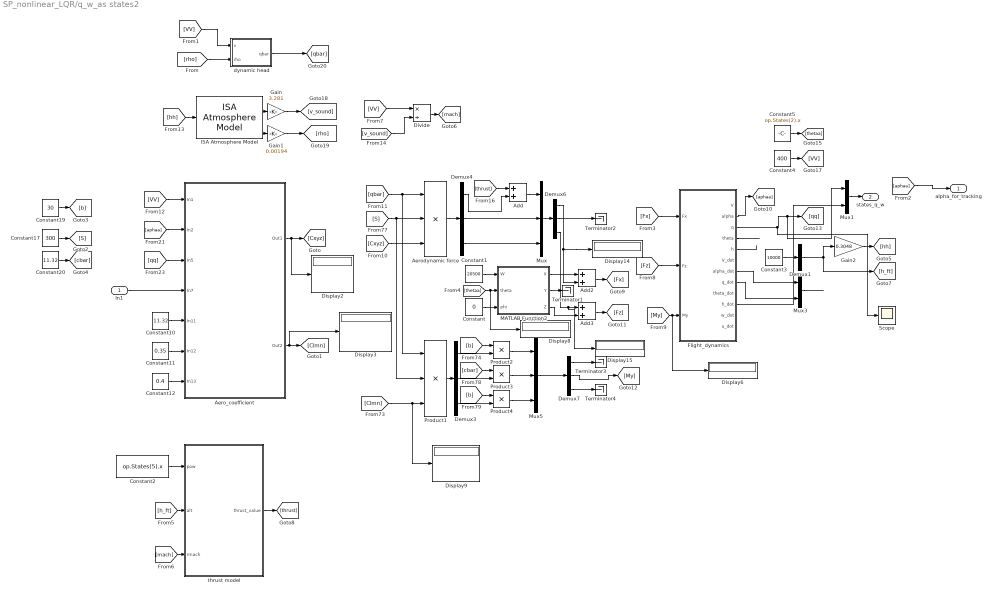
== system SP_nonlinear_LQR/q_w_as states2 ==
  In1 : Inport
  Add : Sum
  Add2 : Sum
  Add3 : Sum
  Aero_coefficient : Subsystem
      mask Display:
      | port_label('input', 1, 'vt')
      | port_label('input', 2, 'alpha')
      | 
      | port_label('input', 3, 'q')
      | 
      | port_label('input', 4, 'el')
      | 
      | 
      | 
      | port_label('input', 5, 'cbar')
      | port_label('input', 6, 'xcgr')
      | port_label('input', 7, 'xcg')
      | port_label('output', 1, 'Cxz')
      | port_label('output', 2, 'Cm')
  "Aerodynamic force " : Product  Inputs=3
  Constant : Constant  Value=0
  Constant1 : Constant  Value=20500
  Constant10 : Constant  Value=11.32
  Constant11 : Constant  Value=0.35
  Constant12 : Constant  Value=0.4
  Constant17 : Constant  Value=300
  Constant19 : Constant  Value=30
  Constant2 : Constant  Value=op.States(5).x
  Constant20 : Constant  Value=11.32
  Constant3 : Constant  Value=10000
  Constant4 : Constant  Value=400
  Constant5 : Constant  Value=op.States(2).x
  Demux1 : Demux  Outputs=1
  Demux{3..4,6..7} (4 alike) : Demux  Outputs=3
  Display{2..3,6,8..9,14..15} (7 alike) : Display
  Divide : Product  Inputs=*/
  Flight_dynamics : Subsystem
  Gain : Gain  Gain=3.281
  Gain1 : Gain  Gain=0.00194
  Gain2 : Gain  Gain=0.3048
  ISA Atmosphere Model : aerolibatmos2/ISA Atmosphere Model  custom=off  g=9.80665  gamma=1.4  R=287.0531  L=0.0065  h_trop=11000  h_strat=20000  rho0=1.225  P0=101325  T0=288.15  h0=0
  MATLAB Function2 : MATLAB Function  TreatAsAtomicUnit=on
  Mux : Mux  Inputs=3
  Mux1 : Mux  Inputs=2
  Mux3 : Mux  Inputs=2
  Mux5 : Mux  Inputs=3
  Product1 : Product  Inputs=3
  Product2 : Product
  Product3 : Product
  Product4 : Product
  Scope : Scope
  Terminator{1..4} (4 alike) : Terminator
  dynamic head : MATLAB Function  TreatAsAtomicUnit=on
  thrust model : MATLAB Function  TreatAsAtomicUnit=on
  alpha_for_tracking : Outport
  states_q_w : Outport  Port=2
  wires:
  [aphaa] -> alpha_for_tracking/1
  Constant5/1 -> [thetaa]
  Constant4/1 -> [VV]
  Constant3/1 -> Demux1/1
  Constant2/1 -> thrust model/1(pow)
  Flight_dynamics/8(q_dot) -> Mux3/2
  Flight_dynamics/7(alpha_dot) -> Mux3/1
  [qq] -> Aero_coefficient/3(In5)
  [aphaa] -> Aero_coefficient/2(In2)
  [VV] -> Aero_coefficient/1(In1)
  Flight_dynamics/5(h) -> ?
  ISA Atmosphere Model/4 -> Gain1/1
  ISA Atmosphere Model/2 -> Gain/1
  [qbar] -> Product1/1, "Aerodynamic force "/1
  In1/1 -> Aero_coefficient/4(In7)
  Product4/1 -> Mux5/3
  Constant10/1 -> Aero_coefficient/5(In11)
  Constant11/1 -> Aero_coefficient/6(In12)
  Mux5/1 -> Demux7/1
  Constant17/1 -> [S]
  Gain1/1 -> [rho]
  Product3/1 -> Mux5/2
  Product2/1 -> Mux5/1
  [VV] -> Divide/1
  [VV] -> dynamic head/1(v)
  Aero_coefficient/1(Out1) -> Display2/1, [Cxyz]
  [rho] -> dynamic head/2(rho)
  Aero_coefficient/2(Out2) -> [Clmn], Display3/1
  Constant20/1 -> [cbar]
  Constant19/1 -> [b]
  Demux1/1 -> Gain2/1, [h_ft]
  [hh] -> ISA Atmosphere Model/1
  Demux4/3 -> Mux/3
  Gain/1 -> [v_sound]
  Divide/1 -> [mach]
  Add/1 -> Mux/1
  Demux4/2 -> Mux/2
  [v_sound] -> Divide/2
  Demux4/1 -> Add/2
  Mux/1 -> Demux6/1
  Constant12/1 -> Aero_coefficient/7(In13)
  Gain2/1 -> [hh]
  dynamic head/1(qbar) -> [qbar]
  thrust model/1(thrust_value) -> [thrust]
  [h_ft] -> thrust model/2(alt)
  [mach] -> thrust model/3(rmach)
  [thrust] -> Add/1
  Demux3/3 -> Product4/2
  [b] -> Product4/1
  "Aerodynamic force "/1 -> Demux4/1
  [Cxyz] -> "Aerodynamic force "/3
  [S] -> "Aerodynamic force "/2, Product1/2
  [Clmn] -> Display9/1, Product1/3
  [b] -> Product2/1
  Product1/1 -> Demux3/1
  Demux3/1 -> Product2/2
  Demux3/2 -> Product3/2
  [cbar] -> Product3/1
  Demux6/3 -> Display15/1, Add3/1
  Demux6/2 -> Terminator2/1
  Demux7/1 -> Terminator3/1
  Demux7/3 -> Terminator4/1
  Constant1/1 -> MATLAB Function2/1(W)
  [thetaa] -> Display8/1, MATLAB Function2/2(theta)
  Constant/1 -> MATLAB Function2/3(phi)
  MATLAB Function2/1(X) -> Add2/1
  Demux6/1 -> Display14/1, Add2/2
  MATLAB Function2/3(Z) -> Add3/2
  MATLAB Function2/2(Y) -> Terminator1/1
  Add2/1 -> [Fx]
  Add3/1 -> [Fz]
  Demux7/2 -> [My]
  [Fx] -> Flight_dynamics/1(Fx)
  [Fz] -> Flight_dynamics/2(Fz)
  [My] -> Flight_dynamics/3(My), Display6/1
  Mux3/1 -> ?
  Flight_dynamics/2(alpha) -> [aphaa]
  Flight_dynamics/3(q) -> Scope/1, Mux1/1, [qq]
  Flight_dynamics/4(theta) -> ?
  Mux1/1 -> states_q_w/1
  Flight_dynamics/10(h_dot) -> Mux1/2

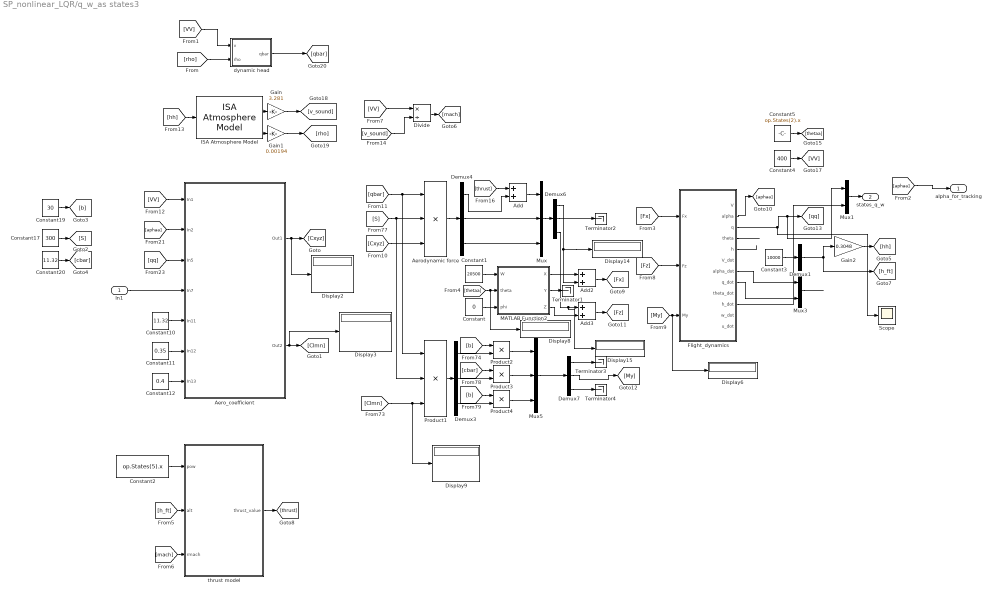
== system SP_nonlinear_LQR/q_w_as states3 ==
  In1 : Inport
  Add : Sum
  Add2 : Sum
  Add3 : Sum
  Aero_coefficient : Subsystem
      mask Display:
      | port_label('input', 1, 'vt')
      | port_label('input', 2, 'alpha')
      | 
      | port_label('input', 3, 'q')
      | 
      | port_label('input', 4, 'el')
      | 
      | 
      | 
      | port_label('input', 5, 'cbar')
      | port_label('input', 6, 'xcgr')
      | port_label('input', 7, 'xcg')
      | port_label('output', 1, 'Cxz')
      | port_label('output', 2, 'Cm')
  "Aerodynamic force " : Product  Inputs=3
  Constant : Constant  Value=0
  Constant1 : Constant  Value=20500
  Constant10 : Constant  Value=11.32
  Constant11 : Constant  Value=0.35
  Constant12 : Constant  Value=0.4
  Constant17 : Constant  Value=300
  Constant19 : Constant  Value=30
  Constant2 : Constant  Value=op.States(5).x
  Constant20 : Constant  Value=11.32
  Constant3 : Constant  Value=10000
  Constant4 : Constant  Value=400
  Constant5 : Constant  Value=op.States(2).x
  Demux1 : Demux  Outputs=1
  Demux{3..4,6..7} (4 alike) : Demux  Outputs=3
  Display{2..3,6,8..9,14..15} (7 alike) : Display
  Divide : Product  Inputs=*/
  Flight_dynamics : Subsystem
  Gain : Gain  Gain=3.281
  Gain1 : Gain  Gain=0.00194
  Gain2 : Gain  Gain=0.3048
  ISA Atmosphere Model : aerolibatmos2/ISA Atmosphere Model  custom=off  g=9.80665  gamma=1.4  R=287.0531  L=0.0065  h_trop=11000  h_strat=20000  rho0=1.225  P0=101325  T0=288.15  h0=0
  MATLAB Function2 : MATLAB Function  TreatAsAtomicUnit=on
  Mux : Mux  Inputs=3
  Mux1 : Mux  Inputs=2
  Mux3 : Mux  Inputs=2
  Mux5 : Mux  Inputs=3
  Product1 : Product  Inputs=3
  Product2 : Product
  Product3 : Product
  Product4 : Product
  Scope : Scope
  Terminator{1..4} (4 alike) : Terminator
  dynamic head : MATLAB Function  TreatAsAtomicUnit=on
  thrust model : MATLAB Function  TreatAsAtomicUnit=on
  alpha_for_tracking : Outport
  states_q_w : Outport  Port=2
  wires:
  [aphaa] -> alpha_for_tracking/1
  Constant5/1 -> [thetaa]
  Constant4/1 -> [VV]
  Constant3/1 -> Demux1/1
  Constant2/1 -> thrust model/1(pow)
  Flight_dynamics/8(q_dot) -> Mux3/2
  Flight_dynamics/7(alpha_dot) -> Mux3/1
  [qq] -> Aero_coefficient/3(In5)
  [aphaa] -> Aero_coefficient/2(In2)
  [VV] -> Aero_coefficient/1(In1)
  Flight_dynamics/5(h) -> ?
  ISA Atmosphere Model/4 -> Gain1/1
  ISA Atmosphere Model/2 -> Gain/1
  [qbar] -> Product1/1, "Aerodynamic force "/1
  In1/1 -> Aero_coefficient/4(In7)
  Product4/1 -> Mux5/3
  Constant10/1 -> Aero_coefficient/5(In11)
  Constant11/1 -> Aero_coefficient/6(In12)
  Mux5/1 -> Demux7/1
  Constant17/1 -> [S]
  Gain1/1 -> [rho]
  Product3/1 -> Mux5/2
  Product2/1 -> Mux5/1
  [VV] -> Divide/1
  [VV] -> dynamic head/1(v)
  Aero_coefficient/1(Out1) -> Display2/1, [Cxyz]
  [rho] -> dynamic head/2(rho)
  Aero_coefficient/2(Out2) -> [Clmn], Display3/1
  Constant20/1 -> [cbar]
  Constant19/1 -> [b]
  Demux1/1 -> Gain2/1, [h_ft]
  [hh] -> ISA Atmosphere Model/1
  Demux4/3 -> Mux/3
  Gain/1 -> [v_sound]
  Divide/1 -> [mach]
  Add/1 -> Mux/1
  Demux4/2 -> Mux/2
  [v_sound] -> Divide/2
  Demux4/1 -> Add/2
  Mux/1 -> Demux6/1
  Constant12/1 -> Aero_coefficient/7(In13)
  Gain2/1 -> [hh]
  dynamic head/1(qbar) -> [qbar]
  thrust model/1(thrust_value) -> [thrust]
  [h_ft] -> thrust model/2(alt)
  [mach] -> thrust model/3(rmach)
  [thrust] -> Add/1
  Demux3/3 -> Product4/2
  [b] -> Product4/1
  "Aerodynamic force "/1 -> Demux4/1
  [Cxyz] -> "Aerodynamic force "/3
  [S] -> "Aerodynamic force "/2, Product1/2
  [Clmn] -> Display9/1, Product1/3
  [b] -> Product2/1
  Product1/1 -> Demux3/1
  Demux3/1 -> Product2/2
  Demux3/2 -> Product3/2
  [cbar] -> Product3/1
  Demux6/3 -> Display15/1, Add3/1
  Demux6/2 -> Terminator2/1
  Demux7/1 -> Terminator3/1
  Demux7/3 -> Terminator4/1
  Constant1/1 -> MATLAB Function2/1(W)
  [thetaa] -> Display8/1, MATLAB Function2/2(theta)
  Constant/1 -> MATLAB Function2/3(phi)
  MATLAB Function2/1(X) -> Add2/1
  Demux6/1 -> Display14/1, Add2/2
  MATLAB Function2/3(Z) -> Add3/2
  MATLAB Function2/2(Y) -> Terminator1/1
  Add2/1 -> [Fx]
  Add3/1 -> [Fz]
  Demux7/2 -> [My]
  [Fx] -> Flight_dynamics/1(Fx)
  [Fz] -> Flight_dynamics/2(Fz)
  [My] -> Flight_dynamics/3(My), Display6/1
  Mux3/1 -> ?
  Flight_dynamics/2(alpha) -> [aphaa]
  Flight_dynamics/3(q) -> Scope/1, Mux1/1, [qq]
  Flight_dynamics/4(theta) -> ?
  Mux1/1 -> states_q_w/1
  Flight_dynamics/10(h_dot) -> Mux1/2

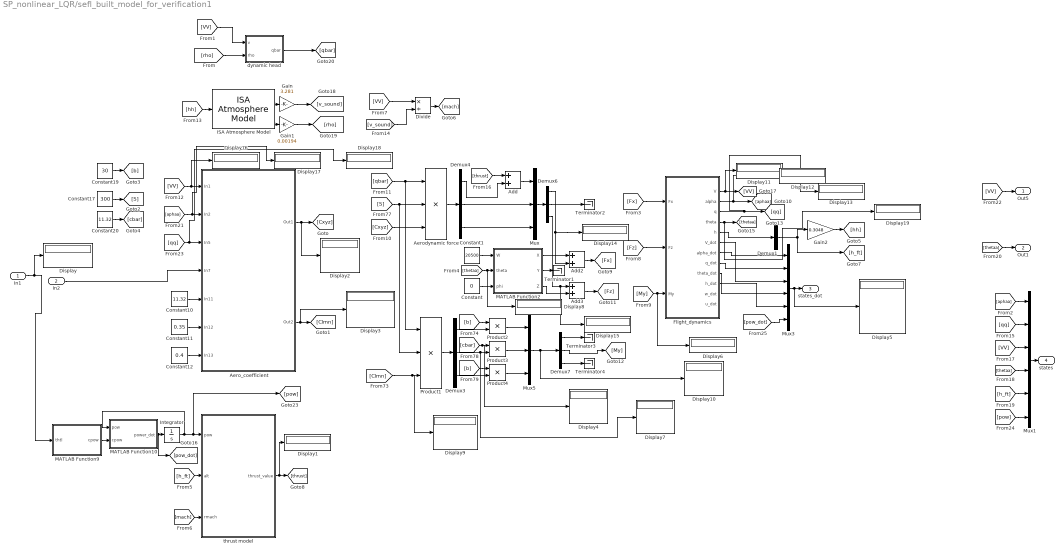
== system SP_nonlinear_LQR/sefl_built_model_for_verification1 ==
  In1 : Inport
  In2 : Inport  Port=2
  Add : Sum
  Add2 : Sum
  Add3 : Sum
  Aero_coefficient : Subsystem
      mask Display:
      | port_label('input', 1, 'vt')
      | port_label('input', 2, 'alpha')
      | 
      | port_label('input', 3, 'q')
      | 
      | port_label('input', 4, 'el')
      | 
      | 
      | 
      | port_label('input', 5, 'cbar')
      | port_label('input', 6, 'xcgr')
      | port_label('input', 7, 'xcg')
      | port_label('output', 1, 'Cxz')
      | port_label('output', 2, 'Cm')
  "Aerodynamic force " : Product  Inputs=3
  Constant : Constant  Value=0
  Constant1 : Constant  Value=20500
  Constant10 : Constant  Value=11.32
  Constant11 : Constant  Value=0.35
  Constant12 : Constant  Value=0.4
  Constant17 : Constant  Value=300
  Constant19 : Constant  Value=30
  Constant20 : Constant  Value=11.32
  Demux1 : Demux  Outputs=1
  Demux{3..4,6..7} (4 alike) : Demux  Outputs=3
  Display{,1..19} (20 alike) : Display
  Divide : Product  Inputs=*/
  Flight_dynamics : Subsystem
  Gain : Gain  Gain=3.281
  Gain1 : Gain  Gain=0.00194
  Gain2 : Gain  Gain=0.3048
  ISA Atmosphere Model : aerolibatmos2/ISA Atmosphere Model  custom=off  g=9.80665  gamma=1.4  R=287.0531  L=0.0065  h_trop=11000  h_strat=20000  rho0=1.225  P0=101325  T0=288.15  h0=0
  Integrator : Integrator  InitialCondition=op.States(5).x
  MATLAB Function10 : MATLAB Function  TreatAsAtomicUnit=on
  MATLAB Function2 : MATLAB Function  TreatAsAtomicUnit=on
  MATLAB Function9 : MATLAB Function  TreatAsAtomicUnit=on
  Mux : Mux  Inputs=3
  Mux1 : Mux  Inputs=6
  Mux3 : Mux  Inputs=6
  Mux5 : Mux  Inputs=3
  Product1 : Product  Inputs=3
  Product2 : Product
  Product3 : Product
  Product4 : Product
  Terminator{1..4} (4 alike) : Terminator
  dynamic head : MATLAB Function  TreatAsAtomicUnit=on
  thrust model : MATLAB Function  TreatAsAtomicUnit=on
  Out5 : Outport
  Out1 : Outport  Port=2
  states_dot : Outport  Port=3
  states : Outport  Port=4
  wires:
  Flight_dynamics/4(theta) -> Display19/1, [thetaa]
  Flight_dynamics/3(q) -> Display13/1, [qq]
  Flight_dynamics/1(V) -> Display11/1, [VV]
  Flight_dynamics/2(alpha) -> Display12/1, [aphaa]
  [VV] -> Out5/1
  Mux3/1 -> Display5/1, states_dot/1
  [pow_dot] -> Mux3/6
  [My] -> Flight_dynamics/3(My), Display6/1
  [Fz] -> Flight_dynamics/2(Fz)
  [Fx] -> Flight_dynamics/1(Fx)
  Demux7/2 -> [My]
  Add3/1 -> [Fz]
  Add2/1 -> [Fx]
  MATLAB Function2/2(Y) -> Terminator1/1
  MATLAB Function2/3(Z) -> Add3/2
  Demux6/1 -> Add2/2, Display14/1
  MATLAB Function2/1(X) -> Add2/1
  Constant/1 -> MATLAB Function2/3(phi)
  [thetaa] -> MATLAB Function2/2(theta), Display8/1
  Constant1/1 -> MATLAB Function2/1(W)
  [thetaa] -> Out1/1
  Demux7/3 -> Terminator4/1
  Demux7/1 -> Terminator3/1
  Demux6/2 -> Terminator2/1
  Demux6/3 -> Add3/1, Display15/1
  [cbar] -> Display4/1, Product3/1
  Demux3/2 -> Display7/1, Product3/2
  Demux3/1 -> Product2/2
  Product1/1 -> Demux3/1
  [b] -> Product2/1
  [Clmn] -> Display9/1, Product1/3
  [S] -> Product1/2, "Aerodynamic force "/2
  [Cxyz] -> "Aerodynamic force "/3
  "Aerodynamic force "/1 -> Demux4/1
  [b] -> Product4/1
  Demux3/3 -> Product4/2
  [thrust] -> Add/1
  MATLAB Function9/1(cpow) -> MATLAB Function10/2(cpow)
  MATLAB Function10/1(power_dot) -> Integrator/1, [pow_dot]
  [mach] -> thrust model/3(rmach)
  Integrator/1 -> MATLAB Function10/1(pow), thrust model/1(pow), [pow]
  In1/1 -> MATLAB Function9/1(thtl), Display/1
  In2/1 -> Aero_coefficient/4(In7)
  [h_ft] -> thrust model/2(alt)
  thrust model/1(thrust_value) -> [thrust], Display1/1
  dynamic head/1(qbar) -> [qbar]
  Gain2/1 -> [hh]
  Constant12/1 -> Aero_coefficient/7(In13)
  Mux/1 -> Demux6/1
  Demux4/1 -> Add/2
  [v_sound] -> Divide/2
  Demux4/2 -> Mux/2
  Add/1 -> Mux/1
  Divide/1 -> [mach]
  Gain/1 -> [v_sound]
  Demux4/3 -> Mux/3
  [hh] -> ISA Atmosphere Model/1
  Demux1/1 -> [h_ft], Gain2/1
  Constant19/1 -> [b]
  Constant20/1 -> [cbar]
  Aero_coefficient/2(Out2) -> Display3/1, [Clmn]
  [rho] -> dynamic head/2(rho)
  Aero_coefficient/1(Out1) -> [Cxyz], Display2/1
  [VV] -> dynamic head/1(v)
  [VV] -> Divide/1
  Product2/1 -> Mux5/1
  Product3/1 -> Mux5/2
  Gain1/1 -> [rho]
  Constant17/1 -> [S]
  Mux5/1 -> Display10/1, Demux7/1
  Constant11/1 -> Aero_coefficient/6(In12)
  Constant10/1 -> Aero_coefficient/5(In11)
  Product4/1 -> Mux5/3
  [qbar] -> "Aerodynamic force "/1, Product1/1
  ISA Atmosphere Model/2 -> Gain/1
  ISA Atmosphere Model/4 -> Gain1/1
  Flight_dynamics/5(h) -> Demux1/1
  [VV] -> Display16/1, Aero_coefficient/1(In1)
  [aphaa] -> Display17/1, Aero_coefficient/2(In2)
  [qq] -> Display18/1, Aero_coefficient/3(In5)
  Flight_dynamics/6(V_dot) -> Mux3/3
  Flight_dynamics/7(alpha_dot) -> Mux3/1
  Flight_dynamics/8(q_dot) -> Mux3/2
  Flight_dynamics/9(theta_dot) -> Mux3/4
  Flight_dynamics/10(h_dot) -> Mux3/5
  [VV] -> Mux1/3
  [qq] -> Mux1/2
  [aphaa] -> Mux1/1
  [thetaa] -> Mux1/4
  [h_ft] -> Mux1/5
  [pow] -> Mux1/6
  Mux1/1 -> states/1

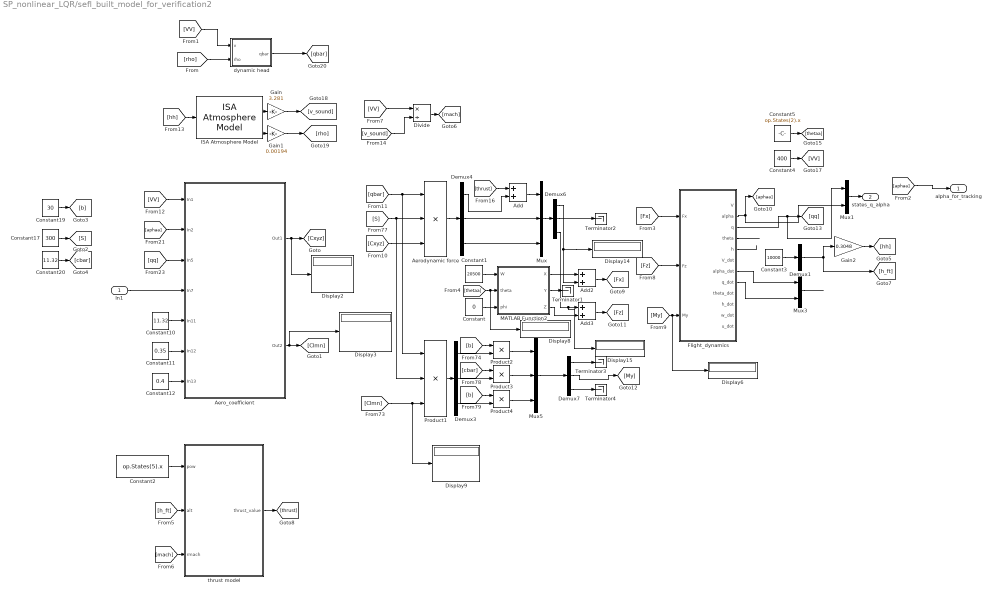
== system SP_nonlinear_LQR/sefl_built_model_for_verification2 ==
  In1 : Inport
  Add : Sum
  Add2 : Sum
  Add3 : Sum
  Aero_coefficient : Subsystem
      mask Display:
      | port_label('input', 1, 'vt')
      | port_label('input', 2, 'alpha')
      | 
      | port_label('input', 3, 'q')
      | 
      | port_label('input', 4, 'el')
      | 
      | 
      | 
      | port_label('input', 5, 'cbar')
      | port_label('input', 6, 'xcgr')
      | port_label('input', 7, 'xcg')
      | port_label('output', 1, 'Cxz')
      | port_label('output', 2, 'Cm')
  "Aerodynamic force " : Product  Inputs=3
  Constant : Constant  Value=0
  Constant1 : Constant  Value=20500
  Constant10 : Constant  Value=11.32
  Constant11 : Constant  Value=0.35
  Constant12 : Constant  Value=0.4
  Constant17 : Constant  Value=300
  Constant19 : Constant  Value=30
  Constant2 : Constant  Value=op.States(5).x
  Constant20 : Constant  Value=11.32
  Constant3 : Constant  Value=10000
  Constant4 : Constant  Value=400
  Constant5 : Constant  Value=op.States(2).x
  Demux1 : Demux  Outputs=1
  Demux{3..4,6..7} (4 alike) : Demux  Outputs=3
  Display{2..3,6,8..9,14..15} (7 alike) : Display
  Divide : Product  Inputs=*/
  Flight_dynamics : Subsystem
  Gain : Gain  Gain=3.281
  Gain1 : Gain  Gain=0.00194
  Gain2 : Gain  Gain=0.3048
  ISA Atmosphere Model : aerolibatmos2/ISA Atmosphere Model  custom=off  g=9.80665  gamma=1.4  R=287.0531  L=0.0065  h_trop=11000  h_strat=20000  rho0=1.225  P0=101325  T0=288.15  h0=0
  MATLAB Function2 : MATLAB Function  TreatAsAtomicUnit=on
  Mux : Mux  Inputs=3
  Mux1 : Mux  Inputs=2
  Mux3 : Mux  Inputs=2
  Mux5 : Mux  Inputs=3
  Product1 : Product  Inputs=3
  Product2 : Product
  Product3 : Product
  Product4 : Product
  Terminator{1..4} (4 alike) : Terminator
  dynamic head : MATLAB Function  TreatAsAtomicUnit=on
  thrust model : MATLAB Function  TreatAsAtomicUnit=on
  alpha_for_tracking : Outport
  states_q_alpha : Outport  Port=2
  wires:
  [aphaa] -> alpha_for_tracking/1
  Constant5/1 -> [thetaa]
  Constant4/1 -> [VV]
  Constant3/1 -> Demux1/1
  Constant2/1 -> thrust model/1(pow)
  Flight_dynamics/8(q_dot) -> Mux3/2
  Flight_dynamics/7(alpha_dot) -> Mux3/1
  [qq] -> Aero_coefficient/3(In5)
  [aphaa] -> Aero_coefficient/2(In2)
  [VV] -> Aero_coefficient/1(In1)
  Flight_dynamics/5(h) -> ?
  ISA Atmosphere Model/4 -> Gain1/1
  ISA Atmosphere Model/2 -> Gain/1
  [qbar] -> Product1/1, "Aerodynamic force "/1
  In1/1 -> Aero_coefficient/4(In7)
  Product4/1 -> Mux5/3
  Constant10/1 -> Aero_coefficient/5(In11)
  Constant11/1 -> Aero_coefficient/6(In12)
  Mux5/1 -> Demux7/1
  Constant17/1 -> [S]
  Gain1/1 -> [rho]
  Product3/1 -> Mux5/2
  Product2/1 -> Mux5/1
  [VV] -> Divide/1
  [VV] -> dynamic head/1(v)
  Aero_coefficient/1(Out1) -> Display2/1, [Cxyz]
  [rho] -> dynamic head/2(rho)
  Aero_coefficient/2(Out2) -> [Clmn], Display3/1
  Constant20/1 -> [cbar]
  Constant19/1 -> [b]
  Demux1/1 -> Gain2/1, [h_ft]
  [hh] -> ISA Atmosphere Model/1
  Demux4/3 -> Mux/3
  Gain/1 -> [v_sound]
  Divide/1 -> [mach]
  Add/1 -> Mux/1
  Demux4/2 -> Mux/2
  [v_sound] -> Divide/2
  Demux4/1 -> Add/2
  Mux/1 -> Demux6/1
  Constant12/1 -> Aero_coefficient/7(In13)
  Gain2/1 -> [hh]
  dynamic head/1(qbar) -> [qbar]
  thrust model/1(thrust_value) -> [thrust]
  [h_ft] -> thrust model/2(alt)
  [mach] -> thrust model/3(rmach)
  [thrust] -> Add/1
  Demux3/3 -> Product4/2
  [b] -> Product4/1
  "Aerodynamic force "/1 -> Demux4/1
  [Cxyz] -> "Aerodynamic force "/3
  [S] -> "Aerodynamic force "/2, Product1/2
  [Clmn] -> Display9/1, Product1/3
  [b] -> Product2/1
  Product1/1 -> Demux3/1
  Demux3/1 -> Product2/2
  Demux3/2 -> Product3/2
  [cbar] -> Product3/1
  Demux6/3 -> Display15/1, Add3/1
  Demux6/2 -> Terminator2/1
  Demux7/1 -> Terminator3/1
  Demux7/3 -> Terminator4/1
  Constant1/1 -> MATLAB Function2/1(W)
  [thetaa] -> Display8/1, MATLAB Function2/2(theta)
  Constant/1 -> MATLAB Function2/3(phi)
  MATLAB Function2/1(X) -> Add2/1
  Demux6/1 -> Display14/1, Add2/2
  MATLAB Function2/3(Z) -> Add3/2
  MATLAB Function2/2(Y) -> Terminator1/1
  Add2/1 -> [Fx]
  Add3/1 -> [Fz]
  Demux7/2 -> [My]
  [Fx] -> Flight_dynamics/1(Fx)
  [Fz] -> Flight_dynamics/2(Fz)
  [My] -> Flight_dynamics/3(My), Display6/1
  Mux3/1 -> ?
  Flight_dynamics/2(alpha) -> Mux1/2, [aphaa]
  Flight_dynamics/3(q) -> Mux1/1, [qq]
  Flight_dynamics/4(theta) -> ?
  Mux1/1 -> states_q_alpha/1
